simulink model "lanedetection_ycbcr"  (R2018a)
settings: Solver=FixedStepAuto  StartTime=0.0  StopTime=inf  RelTol=1e-3  EnableMultiTasking=on
undefined symbols (not defined in the file or in its folder): gray
libraries: visiongeotforms x4, visiontransforms x2, embdlinuxlib x2, dspmtrx3 x2, visiontextngfix x1, visionanalysis x1, visionstatistics x1
settings Model: SimulationMode=external  Creator=ifadmin  LastModifiedBy=ifadmin
settings SolverCC: PositivePriorityOrder=on
settings OptimizationCC: EnhancedBackFolding=on  PassReuseOutputArgsAs=Individual arguments  MaxStackSize=64  OptimizeBlockOrder=speed  DifferentSizesBufferReuse=on  OptimizationCustomize=off
settings DebuggingCC: ParameterTunabilityLossMsg=error
settings HardwareCC: ProdBitPerPointer=32  ProdBitPerSizeT=32  ProdBitPerPtrDiffT=32  ProdLargestAtomicInteger=Long  ProdLargestAtomicFloat=Double  ProdWordSize=32  ProdHWDeviceType=ARM Compatible->ARM Cortex
settings SFSimCC: MATLABDynamicMemAlloc=off
settings RTWCC: SystemTargetFile=ert.tlc  HardwareBoard=Raspberry Pi  TLCOptions="-aInlineSetEventsForThisBaseRateFcn=TLC_FALSE -aSuppressMultiTaskScheduler=TLC_FALSE  -aRateBasedStepFcn=0"  TemplateMakefile=ert_default_tmf  GenerateReport=on  Toolchain=GNU GCC Raspberry Pi  BuildConfiguration=Faster Runs  IncludeHyperlinkInReport=on  LaunchReport=on  GenerateTraceInfo=on  GenerateTraceReport=on  GenerateTraceReportSl=on  GenerateTraceReportSf=on  GenerateTraceReportEml=on
settings CodeAppCC: ForceParamTrailComments=on  IgnoreCustomStorageClasses=off  OperatorAnnotations=on  SimulinkDataObjDesc=on  SFDataObjDesc=on  InsertBlockDesc=on
settings ERTTargetCC: SupportVariableSizeSignals=on

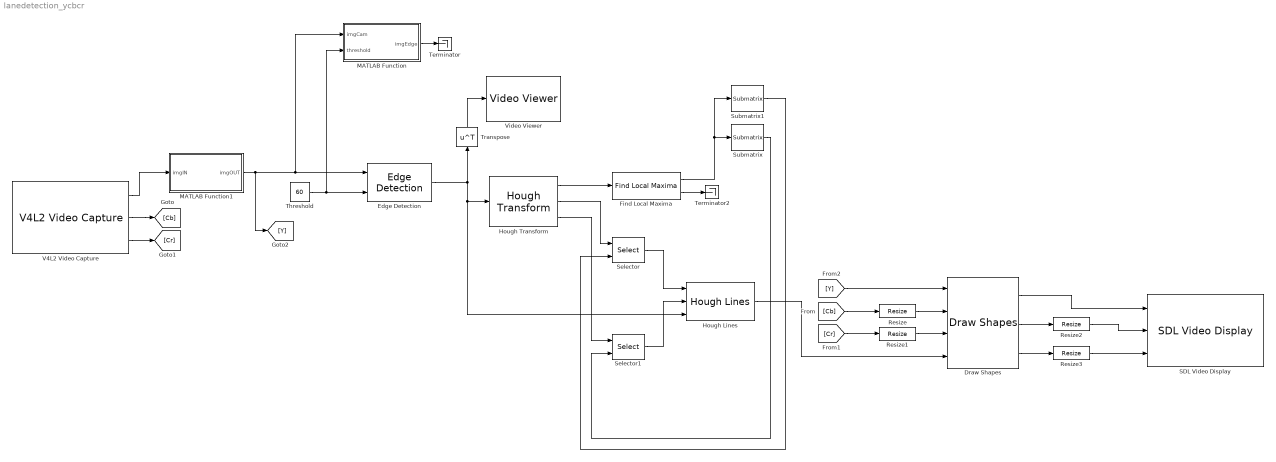
== system lanedetection_ycbcr ==
  Draw Shapes : visiontextngfix/Draw Shapes  shape=Lines  fill=off  lineWidth=2  fillClrSource=Specify via dialog  display=User-specified value  intensity=200  color=[255 000 000]  opacity=0.6  viewport=Entire image  antialiasing=on  inType=Obsolete  imagePorts=Separate color signals  prodOutputMode=Binary point scaling  prodOutputWordLength=32  prodOutputFracLength=14  memoryMode=Specify word length  memoryWordLength=16  memoryFracLength=14  roundingMode=Floor  overflowMode=off
      settings: SourceProductName=Computer Vision System Toolbox  LockScale=on
  Edge Detection : visionanalysis/Edge Detection  method=Roberts  outputType=Binary image  userDefinedThreshold=on  thresholdSource=Input port  threshold=20  thresholdTuning=4  edgeThinning=off  threshold_canny=[0.25 0.60]  autoPercent=70  sigma=1  roundingMode=Floor  overflowMode=off  prodOutputMode=Binary point scaling  prodOutputWordLength=32  prodOutputFracLength=8  prodOutputSlope=2^-8  accumSlope=2^-8  outputSlope=2^-4
      settings: SourceProductName=Computer Vision System Toolbox  SourceProductBaseCode=VP
  Find Local Maxima : visionstatistics/Find Local Maxima  num_peaks=1  nhood_size=[5 7]  src_thresh=Obsolete9b  src_thresh_inuse=Specify via dialog  threshold=10  inputIsHough=on  dt_peak=uint32  isOutVarDim=off  dt_count=uint32
      settings: SourceProductName=Computer Vision System Toolbox  SourceProductBaseCode=VP
  Hough Lines : visiontransforms/Hough Lines  sineCompMethod=Trigonometric function  thetaRes=pi/180  firstCoeffMode=Specify word length  firstCoeffWordLength=16  firstCoeffFracLength=15  prodOutputMode=Binary point scaling  prodOutputWordLength=32  prodOutputFracLength=16  roundingMode=Nearest  overflowMode=on
      settings: SourceProductName=Computer Vision System Toolbox  SourceProductBaseCode=VP  LockScale=on
  Hough Transform : visiontransforms/Hough Transform  theta_res=pi/180  rho_res=1  out_theta_rho=on  outdtmode=single  firstCoeffMode=Binary point scaling  firstCoeffWordLength=16  firstCoeffFracLength=14  secondCoeffMode=Binary point scaling  secondCoeffWordLength=32  secondCoeffFracLength=16  outputMode=Binary point scaling  outputWordLength=16  outputFracLength=0  accumMode=Binary point scaling  accumWordLength=32  accumFracLength=20  prodOutputMode=Binary point scaling  prodOutputWordLength=32  prodOutputFracLength=20  memoryMode=Binary point scaling  memoryWordLength=32  memoryFracLength=16  roundingMode=Nearest  overflowMode=on
      settings: SourceProductName=Computer Vision System Toolbox  SourceProductBaseCode=VP
  MATLAB Function : MATLAB Function  TreatAsAtomicUnit=on
  MATLAB Function1 : MATLAB Function  TreatAsAtomicUnit=on
  Resize : visiongeotforms/Resize  specify=Number of output rows and columns  rfactor=[200 100]  outCols=25  outRows=25  outRowsCols=[320 100]  interp_method=Bilinear  antialias=on  useROI=off  roiFlag=off  prodOutputMode=Binary point scaling  prodOutputWordLength=32  prodOutputFracLength=10  roundingMode=Nearest  overflowMode=on
      settings: SourceProductName=Computer Vision System Toolbox  SourceProductBaseCode=VP
  Resize1 : visiongeotforms/Resize  specify=Number of output rows and columns  rfactor=[320 100]  outCols=25  outRows=25  outRowsCols=[320 100]  interp_method=Bilinear  antialias=on  useROI=off  roiFlag=off  prodOutputMode=Binary point scaling  prodOutputWordLength=32  prodOutputFracLength=10  roundingMode=Nearest  overflowMode=on
      settings: SourceProductName=Computer Vision System Toolbox  SourceProductBaseCode=VP
  Resize2 : visiongeotforms/Resize  specify=Output size as a percentage of input size  rfactor=[50 100]  outCols=25  outRows=25  outRowsCols=[25 35]  interp_method=Bilinear  antialias=on  useROI=off  roiFlag=off  prodOutputMode=Binary point scaling  prodOutputWordLength=32  prodOutputFracLength=10  roundingMode=Nearest  overflowMode=on
      settings: SourceProductName=Computer Vision System Toolbox  SourceProductBaseCode=VP
  Resize3 : visiongeotforms/Resize  specify=Output size as a percentage of input size  rfactor=[50 100]  outCols=25  outRows=25  outRowsCols=[25 35]  interp_method=Bilinear  antialias=on  useROI=off  roiFlag=off  prodOutputMode=Binary point scaling  prodOutputWordLength=32  prodOutputFracLength=10  roundingMode=Nearest  overflowMode=on
      settings: SourceProductName=Computer Vision System Toolbox  SourceProductBaseCode=VP
  SDL Video Display : embdlinuxlib/SDL Video Display  pixelFormat=YCbCr 4:2:2  pixelOrder=Planar  rowMajor=on  blockPlatform=Raspberry Pi
      settings: SourceProductName=Simulink Support Package for Raspberry Pi Hardware  SourceProductBaseCode=RASPPI
  Selector : Selector  InputPortWidth=180  IndexOptions=Index vector (port)  Indices=[1 3]  OutputSizes=1
  Selector1 : Selector  InputPortWidth=671  IndexOptions=Index vector (port)  Indices=[1 3]  OutputSizes=1
  Submatrix : dspmtrx3/Submatrix  RowSpan=All rows  RowStartMode=First  RowStartIndex=1  RowEndMode=Last  RowEndIndex=1  ColSpan=All columns  ColStartMode=First  ColStartIndex=1  ColEndMode=Last  ColEndIndex=1
  Submatrix1 : dspmtrx3/Submatrix  RowSpan=Range of rows  RowStartMode=First  RowStartIndex=1  RowEndMode=Last  RowEndIndex=1  ColSpan=Range of columns  ColStartMode=First  ColStartIndex=1  ColEndMode=Last  ColEndIndex=1
  Terminator : Terminator
  Terminator2 : Terminator
  Threshold : Constant  Value=60  OutDataTypeStr=uint8
  Transpose : Math  Operator=transpose  SaturateOnIntegerOverflow=on
  V4L2 Video Capture : embdlinuxlib/V4L2 Video Capture  m_devName='/dev/video0'  roi=[0, 0, 640, 480]  imSizeSelection=320x240  imSize=[640, 480]  pixelFormat=YCbCr 4:2:2  pixelOrder=Planar  sampleTime=1/10  simOutput=Colorbars  blockPlatform=Raspberry Pi
      settings: SourceProductName=Simulink Support Package for Raspberry Pi Hardware  SourceProductBaseCode=RASPPI
  Video Viewer : VideoViewer  colormapValue=gray(256)  FigPos=[1054 448 842 305]
  wires:
  V4L2 Video Capture/1 -> MATLAB Function1/1(imgIN)
  V4L2 Video Capture/2 -> [Cb]
  V4L2 Video Capture/3 -> [Cr]
  MATLAB Function1/1(imgOUT) -> [Y], Edge Detection/1, MATLAB Function/1(imgCam)
  Transpose/1 -> Video Viewer/1
  Selector1/1 -> Hough Lines/2
  Hough Transform/1 -> Find Local Maxima/1
  Hough Transform/2 -> Selector/1
  Hough Transform/3 -> Selector1/1
  Selector/1 -> Hough Lines/1
  Submatrix1/1 -> Selector/2
  Find Local Maxima/1 -> Submatrix1/1, Submatrix/1
  Find Local Maxima/2 -> Terminator2/1
  Submatrix/1 -> Selector1/2
  Hough Lines/1 -> Draw Shapes/4
  [Y] -> Draw Shapes/1
  [Cb] -> Resize/1
  [Cr] -> Resize1/1
  Draw Shapes/1 -> SDL Video Display/1
  Draw Shapes/2 -> Resize2/1
  Draw Shapes/3 -> Resize3/1
  Threshold/1 -> MATLAB Function/2(threshold), Edge Detection/2
  Resize/1 -> Draw Shapes/2
  Resize1/1 -> Draw Shapes/3
  Resize2/1 -> SDL Video Display/2
  Resize3/1 -> SDL Video Display/3
  Edge Detection/1 -> Hough Lines/3, Hough Transform/1, Transpose/1
  MATLAB Function/1(imgEdge) -> Terminator/1

== matlab function lanedetection_ycbcr/MATLAB Function1 ==
  data: imgIN input uint8 size=[320 240]; imgOUT output uint8 size=[320 100]
function imgOUT   = imgROI(imgIN)

    % imgIN Array von 160x120
    % rectangle('Position',[x,y,w,h])
    
    imgOUT = imgIN(0:319,120:219);

end

== matlab function lanedetection_ycbcr/MATLAB Function ==
  data: imgCam input size=[320 100]; imgEdge output size=[320 100]; threshold input
function imgEdge   = lanedetection(imgCam, threshold)

    % create laplacian filter
    k = [1 2 1; 0 0 0; -1 -2 -1];
    % run sobel
    V = conv2(double(imgCam), k', 'same');
    % filter edges
    imgEdge = V > threshold;

end
